simulink model "Controllerlogic"  (R2017a)
settings: Solver=ode23tb  StartTime=0.0  StopTime=Inf  RelTol=1e-4
libraries: dspnetwork x12, powerlib x8, sps_avr x7, simulink x3, dspstat3 x2, utility x1
Description:
  | Copyright 2008-2016 The MathWorks, Inc.
settings Model: FPTRunName=Active  ExtModeTrigMode=oneshot  ExtModeArmWhenConnect=off  ExtModeAutoUpdateStatusClock=off  Creator=MathWorks  LastModifiedBy=CCRE
settings SolverCC: ZeroCrossAlgorithm=Adaptive
settings DataIOCC: SaveFormat=Array  SignalLoggingSaveFormat=ModelDataLogs  SignalLoggingName=sigsOut  OutputTimes=[0:1/20:10]
settings OptimizationCC: BlockReduction=off  BooleanDataType=off  ExpressionDepthLimit=2147483647  InitFltsAndDblsToZero=on  EfficientMapNaN2IntZero=off  LifeSpan=inf
settings DebuggingCC: UnderspecifiedInitializationDetection=Classic  MergeDetectMultiDrivingBlocksExec=none  CheckExecutionContextPreStartOutputMsg=on  CheckExecutionContextRuntimeOutputMsg=on  SignalResolutionControl=TryResolveAllWithWarning  IgnoredZcDiagnostic=none  MultiTaskDSMMsg=warning  MultiTaskCondExecSysMsg=none  SigSpecEnsureSampleTimeMsg=none  FcnCallInpInsideContextMsg=warning  UnconnectedInputMsg=none  UnconnectedOutputMsg=none  UnconnectedLineMsg=none  StateNameClashWarn=warning  SFUnexpectedBacktrackingDiag=warning  SFNoUnconditionalDefaultTransitionDiag=warning  SFExecutionAtInitializationDiag=none
settings HardwareCC: ProdBitPerPointer=32  ProdBitPerSizeT=32  ProdBitPerPtrDiffT=32  ProdLargestAtomicFloat=None  ProdIntDivRoundTo=Undefined  ProdEndianess=Unspecified  ProdWordSize=32  ProdHWDeviceType=Specified  TargetUnknown=on
settings ModelReferenceCC: PropagateSignalLabelsOutOfModel=off
settings GRTTargetCC: TargetFcnLib=ansi_tfl_tmw.mat  TargetLangStandard=C89/C90 (ANSI)  GeneratePreprocessorConditionals=Disable all  CombineOutputUpdateFcns=off  GRTInterface=on
settings ConfigComp: CovMetricSettings=dw  CovHtmlReporting=on  CovSaveCumulativeToWorkspaceVar=on  CovSaveSingleToWorkspaceVar=on  CovExternalEMLEnable=off  CovSFcnEnable=off

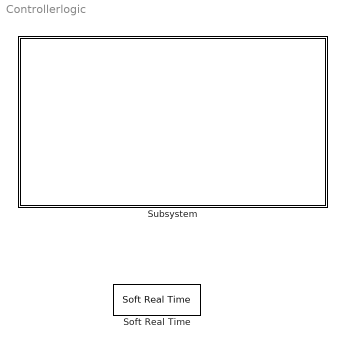
== system Controllerlogic ==
  Soft Real Time : utility/Soft Real Time  x=1
  Subsystem : Subsystem

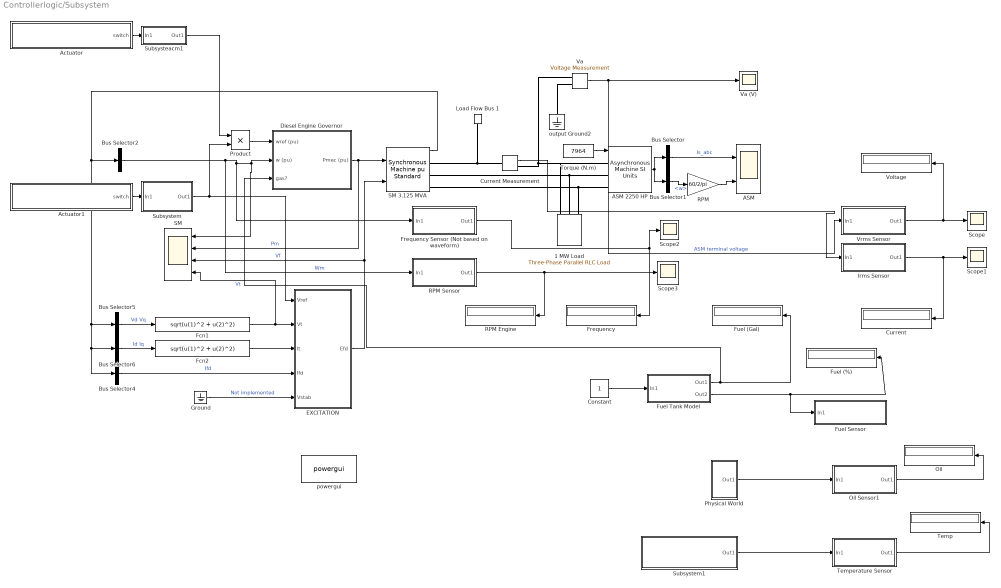
== system Controllerlogic/Subsystem ==
  1 MW Load : powerlib/Elements/Three-Phase Parallel RLC Load  LConnTagsString=A|B|C  Configuration=Y (grounded)  NominalVoltage=2400  Vabc=[1e3 1e3 1e3]  Vabcp=[1e3 1e3 1e3]  NominalFrequency=60  UnbalancedPower=off  ActivePower=1e+006  InductivePower=0  CapacitivePower=0  Pabc=[10e3 9e3 11e3]  QLabc=[100 90 110]  QCabc=[100 90 110]  Pabcp=[10e3 9e3 11e3]  QLabcp=[100 90 110]  QCabcp=[100 90 110]  Measurements=None  LoadType=constant Z
  ASM : Scope  NumInputPorts=2
  ASM 2250 HP : powerlib/Machines/Asynchronous Machine SI Units  RotorType=Squirrel-cage  PresetModel=No  MechanicalLoad=Torque Tm  ShowDetailedParameters=on  ReferenceFrame=Rotor  Units=SI  MeasurementBus=on  NominalParameters=[ 2250*746, 2400, 60 ]  Stator=[ 0.029 0.226/377]  Rotor=[ 0.022 0.226/377]  Cage1=[ 0.022 0.226/377]  Cage2=[ 0.022 0.226/377]  Lm=13.04/377  Mechanical=[ 63.87 0 2]  PolePairs=2  InitialConditions=[0 0 0 0 0 0 0 0]  SimulateSaturation=off  Saturation=[14.03593122, 27.81365428, 53.79336849, 72.68890987, 97.98006896, 148.6815601, 215.7428561, 302.9841135, 428.7778367 ; 230, 322, 414, 460, 506, 552, 598, 644, 690]  LoadFlowParameters=1492000  TsPowergui=0  TsBlock=-1  IterativeModel=Trapezoidal non iterative  IterativeDiscreteModel=Trapezoidal non iterative  Pmec=1.492e+006
  Actuator : Subsystem
  Actuator1 : Subsystem
  Bus Selector : BusSelector  OutputSignals=ias,ibs,ics  OutputAsBus=on
  Bus Selector1 : BusSelector  OutputSignals=w
  Bus Selector2 : BusSelector  OutputSignals="Mechanical.Rotor speed  wm  (pu)"  OutputAsBus=on
  Bus Selector4 : BusSelector  OutputSignals="dq0 components.Field current  ifd (pu)"  OutputAsBus=on
  Bus Selector5 : BusSelector  OutputSignals="dq0 components.Stator voltage  vd (pu),dq0 components.Stator voltage  vq (pu)"  OutputAsBus=on
  Bus Selector6 : BusSelector  OutputSignals="dq0 components.Stator current  id (pu),dq0 components.Stator current  iq (pu)"  OutputAsBus=on
  Constant : Constant
  Current : Display
  Current Measurement : powerlib/Measurements/Current Measurement  PhasorSimulation=off  OutputType=Complex  PSBequivalent=0
  "Diesel Engine Governor " : Subsystem  mask(Diesel Engine & Governor){K=1, Tr=[0.01 0.02 0.2], Ta=[0.25 0.009 0.0384], Tlim=[0 1.1], Td=0.024, Pm0=0}
      mask prompts: K "Regulator gain K:"; Tr "Regulator time constants [T1 T2 T3 ] (s) :"; Ta "Actuator time constants [T4 T5 T6] (s) :"; Tlim "Torque limits [Tmin Tmax] (pu) :"; Td "Engine time delay Td (s) :"; Pm0 "Initial value of mechanical power  Pm0 (pu) :"
      mask help:
      | This block implements a diesel engine and governor system:
      | 1st and 2nd inputs: Desired and actual speed (pu)
      | Output: Diesel engine mechanical power.Motor inertia should be combined with generator.
      | Controller transfer function:
      |      Hc=K.(1+T3.s)/(1+T1.s+T1.T2.s^2)
      | Actuator transfer function :
      |      Ha= (1+T4.s) / [ (s (1+T5.s)(1+T6.s) ]
      | Motor :
      |      Time delay Td
      |
      | (See reference in Tutorial Session 5)
  EXCITATION : Subsystem  Variant=on  OverrideUsingVariant=Variant1
      settings: AttributesFormatString=%<BlockChoice>
  Fcn1 : Fcn  Expr=sqrt(u(1)^2 + u(2)^2)
  Fcn2 : Fcn  Expr=sqrt(u(1)^2 + u(2)^2)
  Frequency : Display
  Frequency Sensor (Not based on waveform) : Subsystem
  Fuel (%) : Display
  Fuel (Gal) : Display
  Fuel Sensor : Subsystem
  Fuel Tank Model : Subsystem
  Ground : Ground
  Irms Sensor : Subsystem
  Load Flow Bus 1 : powerlib/Measurements/Load Flow Bus  LConnTagsString=a  Phases=single  Connectors=on one side  ID=B2  Vbase=2.4e3  Vref=1  Vangle=0  VLF=1  VLFb=1  VLFc=1  angleLF=-31.89  angleLFb=0  angleLFc=0
      settings: AttributesFormatString=%<ID>\n%<Vbase>V\n%<VLF>pu\n%<angleLF>deg.  SourceProductName=Simscape Power Systems
  Oil : Display
  Oil Sensor1 : Subsystem
  Physical World : Subsystem
  Product : Product
  RPM : Gain  Gain=60/2/pi  SaturateOnIntegerOverflow=on  OutDataTypeStr=Inherit: Same as input  ParamDataTypeStr=Inherit: Same as input
  RPM Engine : Display
  RPM Sensor : Subsystem
  SM : Scope  NumInputPorts=4
  SM 3.125 MVA : powerlib/Machines/Synchronous Machine pu Standard  PresetModel=No  MechanicalLoad=Mechanical power Pm  ShowDetailedParameters=on  RotorType=Salient-pole  Units=per unit standard parameters  MeasurementBus=off  NominalParameters="[ 3.125e6  2400  60]"  Reactances1=[ 31 32 33 34 35 36 37 ]  Reactances2=[ 1.56, 0.296, 0.177, 1.06, 0.177, 0.052 ]  dAxisTimeConstants=Short-circuit  qAxisTimeConstants=Open-circuit  TimeConstants1=[]  TimeConstants2=[]  TimeConstants3=[]  TimeConstants4=[]  TimeConstants5=[ 3.7, 0.05, 0.05 ]  TimeConstants6=[ 8.0, 0.03, 0.3371, 0.0295 ]  TimeConstants7=[0.024 0.006 0.006]  TimeConstants8=[]  StatorResistance=0.0036  Mechanical="[ 1.07  0 2]"  PolePairs=2  InitialConditions=[0 0 0 0 0 0 0 0 1]  SetSaturation=off  Saturation=[0.211 0.418 1.0 1.25 1.72 3.35 ;0.25 0.50 1.0 1.1 1.2 1.4]  LoadFlowParameters=[1 0 0 0]  TsPowergui=0  TsBlock=-1  IterativeModel=Trapezoidal non iterative  IterativeDiscreteModel=Trapezoidal non iterative  BusType=PV  Pref=0  Qref=0  Qmin=-Inf  Qmax=Inf  PLF=0  QLF=0
      settings: AttributesFormatString=\n\n  SourceProductName=Simscape Power Systems
  Scope{,1..3} (4 alike) : Scope
  Subsysteacm1 : Subsystem
  Subsystem : Subsystem
  Subsystem1 : Subsystem
  Temp : Display
  Temperature Sensor : Subsystem
  Torque (N.m) : Constant  Value=7964
  Va : powerlib/Measurements/Voltage Measurement  Tag=PoWeRsYsTeMmEaSuReMeNt  PhasorSimulation=off  OutputType=Magnitude  PSBequivalent=0
  Va (V) : Scope
  Voltage : Display
  Vrms Sensor : Subsystem
  output Ground2 : powerlib/Elements/Ground  LConnTagsString=a
  powergui : powerlib/powergui  Priority=2  SimulationMode=Continuous  SampleTime=50e-6  frequency=60  Iterations=50  frequencyindice=60  Pbase=1e6  ErrMax=0.0001  UnitsV=kV  UnitsW=MW  buscounter=0  FunctionMessages=off  echomessages=off  EnableUseOfTLC=off  CurrentSourceSwitches=off  DisableSnubberDevices=on  DisableRonSwitches=off  DisableVfSwitches=off  DisplayEquations=off  SolverType=Tustin  Interpol=off  ExternalGateDelay=off  methode=off  Ts=0  x0status=blocks  SPID=on  SwTol=0  HookPort=off  RestoreLinks=warning  ResistiveCurrentMeasurement=off  Frange=logspace(0,3,50)  Ylog=off  Xlog=off  ShowGrid=off  save=off  variable=ZData  structure=0  ZoomFFT=on  StartTime=0.0  cycles=2  DisplayStyle=off  fundamental=60  FreqAxis=off  MaxFrequency=1000  frequencyindicesteady=1  RmsSteady=1  display=off
  wires:
  "Diesel Engine Governor "/1(Pmec (pu)) -> SM/2, SM 3.125 MVA/1  "Pm"
  Bus Selector4/1 -> EXCITATION/4(Ifd)  "Ifd"
  Bus Selector5/1 -> Fcn1/1  "Vd Vq"
  Bus Selector2/1 -> RPM Sensor/1(In1), Frequency Sensor (Not based on waveform)/1(In1), SM/1, "Diesel Engine Governor "/2(w (pu))  "Wm"
  Bus Selector1/1 -> RPM/1  "<w>"
  Fcn1/1 -> SM/4, EXCITATION/2(Vt)  "Vt"
  RPM/1 -> ASM/2
  Bus Selector6/1 -> Fcn2/1  "Id Iq"
  Ground/1 -> EXCITATION/5(Vstab)  "Not implemented"
  Bus Selector/1 -> ASM/1  "Is_abc"
  Fcn2/1 -> EXCITATION/3(It)
  EXCITATION/1(Efd) -> SM 3.125 MVA/2, SM/3  "Vf"
  SM 3.125 MVA/1 -> Bus Selector5/1, Bus Selector6/1, Bus Selector4/1, Bus Selector2/1
  Vrms Sensor/1(Out1) -> Voltage/1, Scope/1
  Irms Sensor/1(Out1) -> Current/1, Scope1/1
  Va/1 -> Vrms Sensor/1(In1), Va (V)/1  "ASM terminal voltage"
  Current Measurement/1 -> Irms Sensor/1(In1)
  ASM 2250 HP/1 -> Bus Selector/1, Bus Selector1/1
  Torque (N.m)/1 -> ASM 2250 HP/1
  RPM Sensor/1(Out1) -> Scope3/1, RPM Engine/1
  Frequency Sensor (Not based on waveform)/1(Out1) -> Scope2/1, Frequency/1
  Constant/1 -> Fuel Tank Model/1(In1)
  Fuel Tank Model/2(Out2) -> Fuel Sensor/1(In1), Fuel (%)/1
  Product/1 -> "Diesel Engine Governor "/1(wref (pu))
  Oil Sensor1/1(Out1) -> Oil/1
  Subsystem/1(Out1) -> EXCITATION/1(Vref), Product/2
  Actuator1/1("switch ") -> Subsystem/1(In1)
  Temperature Sensor/1(Out1) -> Temp/1
  Actuator/1("switch ") -> Subsysteacm1/1(In1)
  Subsysteacm1/1(Out1) -> Product/1
  Fuel Tank Model/1(Out1) -> "Diesel Engine Governor "/3(gas?), Fuel (Gal)/1
  Physical World/1(Out1) -> Oil Sensor1/1(In1)
  Subsystem1/1(Out1) -> Temperature Sensor/1(In1)
  connections:
  SM 3.125 MVA/RConn3 -- ASM 2250 HP/LConn3 -- 1 MW Load/LConn3
  ASM 2250 HP/LConn1 -- 1 MW Load/LConn1 -- Current Measurement/RConn1 -- Va/LConn1
  output Ground2/LConn1 -- Va/LConn2
  SM 3.125 MVA/RConn2 -- ASM 2250 HP/LConn2 -- 1 MW Load/LConn2
  Load Flow Bus 1/LConn1 -- Current Measurement/LConn1 -- SM 3.125 MVA/RConn1

== system Controllerlogic/Subsystem/Actuator ==
  note: Pump Control
  Display : Display
  Pump If : If  IfExpression=u1 == 0
  Pump Value Conversion : Subsystem  TreatAsAtomicUnit=on
  Terminator : Terminator
  Terminator2 : Terminator
  UDP Receive1 : dspnetwork/UDP Receive  localURL='0.0.0.0'  localPort=10006  remoteURL='0.0.0.0'  remotePort=-1  recvBufferSize=8192  dims=1  signalDatatype=uint8  isVarSize=off  showBlockingTime=on  blockingTime=0  sampletime=0.01  blockPlatform=LINUX
  "switch " : Outport  PortDimensions=1
  wires:
  Pump If/1 -> Terminator/1
  Pump If/2 -> Pump Value Conversion/Action
  UDP Receive1/1 -> Pump Value Conversion/1(P_ASCII), Pump If/1
  Pump Value Conversion/1(P_Val) -> "switch "/1, Display/1
  UDP Receive1/2 -> Terminator2/1

== system Controllerlogic/Subsystem/Actuator1 ==
  note: Pump Control
  Display : Display
  Pump If : If  IfExpression=u1 == 0
  Pump Value Conversion : Subsystem  TreatAsAtomicUnit=on
  Terminator : Terminator
  Terminator2 : Terminator
  UDP Receive1 : dspnetwork/UDP Receive  localURL='0.0.0.0'  localPort=10007  remoteURL='0.0.0.0'  remotePort=-1  recvBufferSize=8192  dims=1  signalDatatype=uint8  isVarSize=off  showBlockingTime=on  blockingTime=0  sampletime=0.01  blockPlatform=LINUX
  "switch " : Outport  PortDimensions=1
  wires:
  Pump If/1 -> Terminator/1
  Pump If/2 -> Pump Value Conversion/Action
  UDP Receive1/1 -> Pump Value Conversion/1(P_ASCII), Pump If/1
  Pump Value Conversion/1(P_Val) -> "switch "/1, Display/1
  UDP Receive1/2 -> Terminator2/1

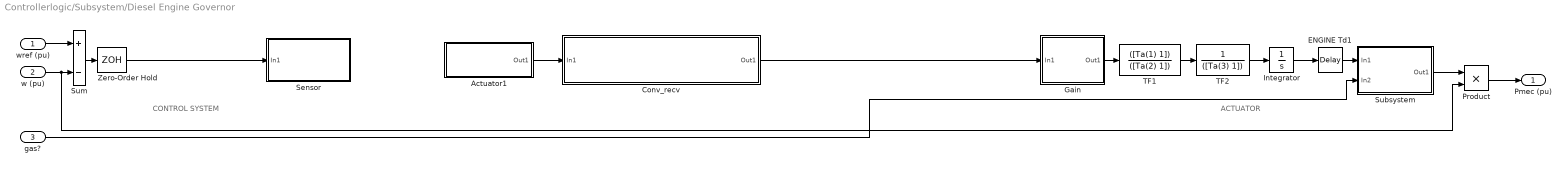
== system Controllerlogic/Subsystem/Diesel Engine Governor  ==
  note: ACTUATOR
  note: CONTROL SYSTEM
  wref (pu) : Inport
  w (pu) : Inport  Port=2
  gas? : Inport  Port=3
  Actuator1 : Subsystem
  Conv_recv : Subsystem
  ENGINE Td1 : TransportDelay  DelayTime=Td  InitialOutput=Pm0
  Gain : Subsystem
  Integrator : Integrator  InitialCondition=Pm0  LimitOutput=on  UpperSaturationLimit=Tlim(2)  LowerSaturationLimit=Tlim(1)
  Product : Product  SaturateOnIntegerOverflow=on  InputSameDT=on  OutDataTypeStr=Inherit: Same as first input
  Sensor : Subsystem
  Subsystem : Subsystem
  Sum : Sum  Inputs=+-  SaturateOnIntegerOverflow=on  InputSameDT=on  OutDataTypeStr=Inherit: Same as first input
  TF1 : TransferFcn  Numerator=([Ta(1) 1])  Denominator=([Ta(2) 1])
  TF2 : TransferFcn  Numerator=1  Denominator=([Ta(3) 1])
  Zero-Order Hold : ZeroOrderHold  SampleTime=.02
  Pmec (pu) : Outport  InitialOutput=0
  wires:
  Product/1 -> Pmec (pu)/1
  wref (pu)/1 -> Sum/1
  w (pu)/1 -> Sum/2, Product/2
  TF1/1 -> TF2/1
  Sum/1 -> Zero-Order Hold/1
  gas?/1 -> Subsystem/2(In2)
  TF2/1 -> Integrator/1
  Integrator/1 -> ENGINE Td1/1
  Subsystem/1(Out1) -> Product/1
  ENGINE Td1/1 -> Subsystem/1(In1)
  Conv_recv/1(Out1) -> Gain/1(In1)
  Gain/1(Out1) -> TF1/1
  Zero-Order Hold/1 -> Sensor/1(In1)
  Actuator1/1(Out1) -> Conv_recv/1(In1)

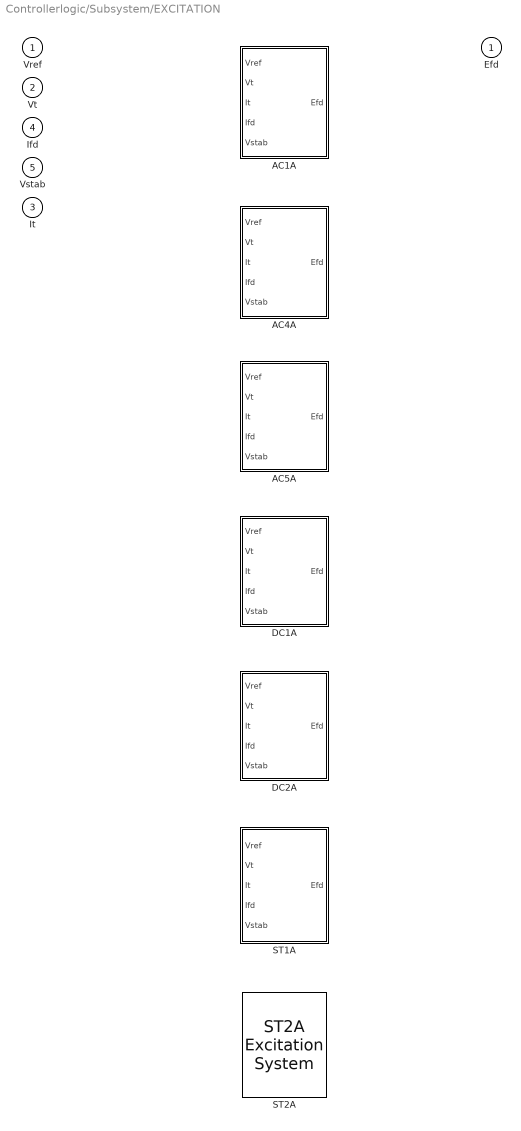
== system Controllerlogic/Subsystem/EXCITATION ==
  Vref : Inport
  Vt : Inport  Port=2
  It : Inport  Port=3
  Ifd : Inport  Port=4
  Vstab : Inport  Port=5
  AC1A : Subsystem  VariantControl=Variant1
  AC4A : Subsystem  VariantControl=Variant2
  AC5A : Subsystem  VariantControl=Variant3
  DC1A : Subsystem  VariantControl=Variant4
  DC2A : Subsystem  VariantControl=Variant5
  ST1A : Subsystem  VariantControl=Variant6
  ST2A : sps_avr/ST2A Excitation System  VariantControl=Variant7  Tr=20e-3  KaTa=[120 0.15]  VRminmax=[0 1.0]  KfTf=[0.05 1.0]  KeTe=[1.0 0.5]  KI=8.0  Kp=4.88  Xd=1.56  Kc=1.82  v0=[1,1.42734]  I0=0.2739  TsBlock=-2
      settings: SourceProductName=Simscape Power Systems  SourceProductBaseCode=PS
  Efd : Outport

== system Controllerlogic/Subsystem/Frequency Sensor (Not based on waveform) ==
  In1 : Inport
  Downsample : DownSample  N=100  RateOptions=Allow multirate processing
  Gain : Gain  Gain=6000
  UDP Send : dspnetwork/UDP Send  remoteURL='192.168.56.101'  remotePort=10003  localURL='255.255.255.255'  localPortSource=Automatically determine  localPort=-1  sampletime=-1  blockPlatform=LINUX  separateLengthPort=0
  Zero-Order Hold : ZeroOrderHold  SampleTime=.001
  Out1 : Outport
  wires:
  In1/1 -> Zero-Order Hold/1
  Zero-Order Hold/1 -> Gain/1
  Downsample/1 -> UDP Send/1, Out1/1
  Gain/1 -> Downsample/1

== system Controllerlogic/Subsystem/Fuel Sensor ==
  In1 : Inport
  Rate Transition : RateTransition
  UDP Send : dspnetwork/UDP Send  remoteURL='192.168.56.101'  remotePort=10005  localURL='255.255.255.255'  localPortSource=Automatically determine  localPort=-1  sampletime=-1  blockPlatform=LINUX  separateLengthPort=0
  Zero-Order Hold1 : ZeroOrderHold  SampleTime=0.1
  Zero-Order Hold2 : ZeroOrderHold  SampleTime=0.01
  wires:
  Rate Transition/1 -> Zero-Order Hold1/1
  Zero-Order Hold1/1 -> UDP Send/1
  Zero-Order Hold2/1 -> Rate Transition/1
  In1/1 -> Zero-Order Hold2/1

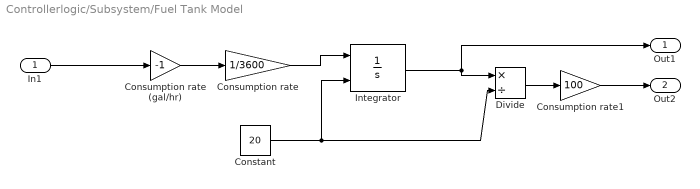
== system Controllerlogic/Subsystem/Fuel Tank Model ==
  In1 : Inport
  Constant : Constant  Value=20
  Consumption rate : Gain  Gain=1/3600
  Consumption rate (gal/hr) : Gain  Gain=-1
  Consumption rate1 : Gain  Gain=100
  Divide : Product  Inputs=*/
  Integrator : Integrator  InitialConditionSource=external  InitialCondition=20  LimitOutput=on  UpperSaturationLimit=20  LowerSaturationLimit=0
  Out1 : Outport
  Out2 : Outport  Port=2
  wires:
  In1/1 -> Consumption rate (gal/hr)/1
  Constant/1 -> Divide/2, Integrator/2
  Integrator/1 -> Divide/1, Out1/1
  Consumption rate1/1 -> Out2/1
  Divide/1 -> Consumption rate1/1
  Consumption rate (gal/hr)/1 -> Consumption rate/1
  Consumption rate/1 -> Integrator/1

== system Controllerlogic/Subsystem/Irms Sensor ==
  In1 : Inport
  Downsample : DownSample  N=100  RateOptions=Allow multirate processing
  RMS : dspstat3/RMS  run=on  directionMode=Entire input  dimension=1  reset_popup=None
  UDP Send : dspnetwork/UDP Send  remoteURL='192.168.56.101'  remotePort=10002  localURL='255.255.255.255'  localPortSource=Automatically determine  localPort=-1  sampletime=-1  blockPlatform=LINUX  separateLengthPort=0
  Zero-Order Hold : ZeroOrderHold  SampleTime=.001
  Out1 : Outport
  wires:
  In1/1 -> Zero-Order Hold/1
  RMS/1 -> Downsample/1
  Zero-Order Hold/1 -> RMS/1
  Downsample/1 -> Out1/1, UDP Send/1

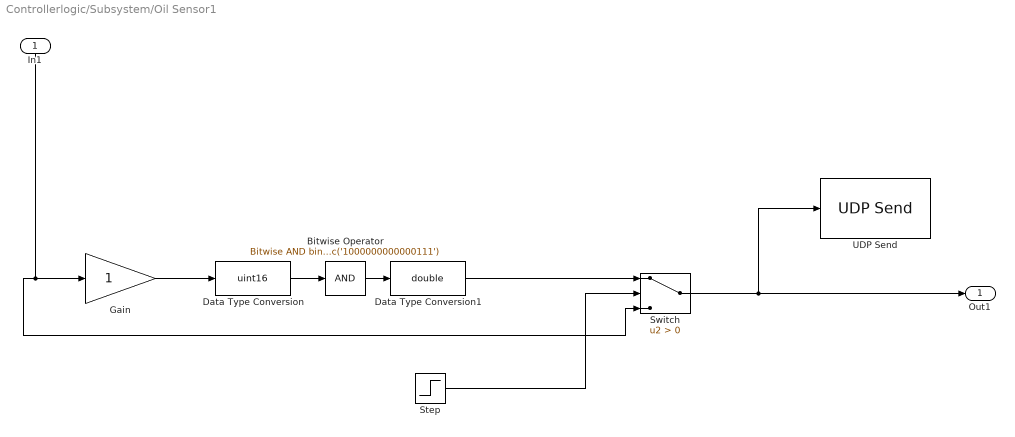
== system Controllerlogic/Subsystem/Oil Sensor1 ==
  In1 : Inport
  Bitwise Operator : simulink/Logic and Bit Operations/Bitwise Operator  logicop=AND  UseBitMask=on  BitMask=bin2dec('1000000000000111')  BitMaskRealWorld=Stored Integer
  Data Type Conversion : DataTypeConversion  OutDataTypeStr=uint16
  Data Type Conversion1 : DataTypeConversion  OutDataTypeStr=double
  Gain : Gain
  Step : Step  SampleTime=0
  Switch : Switch  Criteria=u2 > Threshold
  UDP Send : dspnetwork/UDP Send  remoteURL='192.168.56.101'  remotePort=10008  localURL='255.255.255.255'  localPortSource=Automatically determine  localPort=-1  sampletime=-1  blockPlatform=LINUX  separateLengthPort=0
  Out1 : Outport
  wires:
  In1/1 -> Gain/1, Switch/3
  Bitwise Operator/1 -> Data Type Conversion1/1
  Gain/1 -> Data Type Conversion/1
  Data Type Conversion/1 -> Bitwise Operator/1
  Switch/1 -> UDP Send/1, Out1/1
  Data Type Conversion1/1 -> Switch/1
  Step/1 -> Switch/2

== system Controllerlogic/Subsystem/Physical World ==
  Constant1 : Constant  Value=10
  Constant2 : Constant  Value=50
  Manual Switch : ManualSwitch
  Out1 : Outport
  wires:
  Constant2/1 -> Manual Switch/1
  Constant1/1 -> Manual Switch/2
  Manual Switch/1 -> Out1/1

== system Controllerlogic/Subsystem/RPM Sensor ==
  In1 : Inport
  Downsample : DownSample  N=100  RateOptions=Allow multirate processing
  Gain : Gain  Gain=3600
  UDP Send : dspnetwork/UDP Send  remoteURL='192.168.56.101'  remotePort=10004  localURL='255.255.255.255'  localPortSource=Automatically determine  localPort=-1  sampletime=-1  blockPlatform=LINUX  separateLengthPort=0
  Zero-Order Hold : ZeroOrderHold  SampleTime=.001
  Out1 : Outport
  wires:
  In1/1 -> Zero-Order Hold/1
  Zero-Order Hold/1 -> Gain/1
  Downsample/1 -> Out1/1, UDP Send/1
  Gain/1 -> Downsample/1

== system Controllerlogic/Subsystem/Subsysteacm1 ==
  In1 : Inport
  Switch : Switch  Criteria=u2 > Threshold
  wref (pu) : Constant  Value=50/60
  wref (pu)1 : Constant
  Out1 : Outport
  wires:
  wref (pu)/1 -> Switch/1
  In1/1 -> Switch/2
  Switch/1 -> Out1/1
  wref (pu)1/1 -> Switch/3

== system Controllerlogic/Subsystem/Subsystem ==
  In1 : Inport
  Subtract : Sum  Inputs=+-
  "Vtref (pu) " : Constant
  Out1 : Outport
  wires:
  Subtract/1 -> Out1/1
  In1/1 -> Subtract/2
  "Vtref (pu) "/1 -> Subtract/1

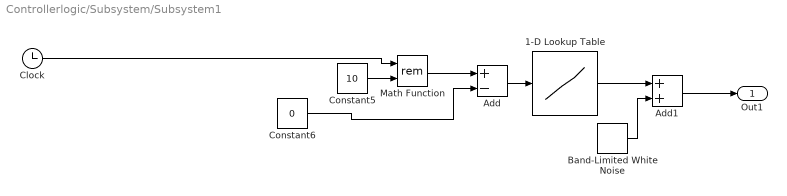
== system Controllerlogic/Subsystem/Subsystem1 ==
  1-D Lookup Table : Lookup_n-D  NumberOfTableDimensions=1  BreakpointsForDimension1=[0 1 2 3 4 5 6 7 8 9 10]  Table=[95 160 95 110 180 110 220 150 110 220 100]  InternalRulePriority=Speed  RndMeth=Simplest  InputSameDT=on
  Add : Sum  Inputs=+-
  Add1 : Sum
  Band-Limited White Noise : simulink/Sources/Band-Limited White Noise  Cov=[0.3]  Ts=0.02  seed=[23341]
  Clock : Clock
  Constant5 : Constant  Value=10
  Constant6 : Constant  Value=0
  Math Function : Math  Operator=rem  SaturateOnIntegerOverflow=on
  Out1 : Outport
  wires:
  Band-Limited White Noise/1 -> Add1/2
  Add/1 -> 1-D Lookup Table/1
  Constant6/1 -> Add/2
  Constant5/1 -> Math Function/2
  Math Function/1 -> Add/1
  Clock/1 -> Math Function/1
  Add1/1 -> Out1/1
  1-D Lookup Table/1 -> Add1/1

== system Controllerlogic/Subsystem/Temperature Sensor ==
  In1 : Inport
  Downsample : DownSample  N=100  RateOptions=Allow multirate processing
  Gain : Gain
  HW Trojan : Subsystem
  UDP Send : dspnetwork/UDP Send  remoteURL='192.168.56.101'  remotePort=10009  localURL='255.255.255.255'  localPortSource=Automatically determine  localPort=-1  sampletime=-1  blockPlatform=LINUX  separateLengthPort=0
  Zero-Order Hold : ZeroOrderHold  SampleTime=.001
  Out1 : Outport
  wires:
  In1/1 -> Zero-Order Hold/1
  Zero-Order Hold/1 -> Gain/1
  Downsample/1 -> HW Trojan/1(In1)
  Gain/1 -> Downsample/1
  HW Trojan/1(Out1) -> Out1/1, UDP Send/1

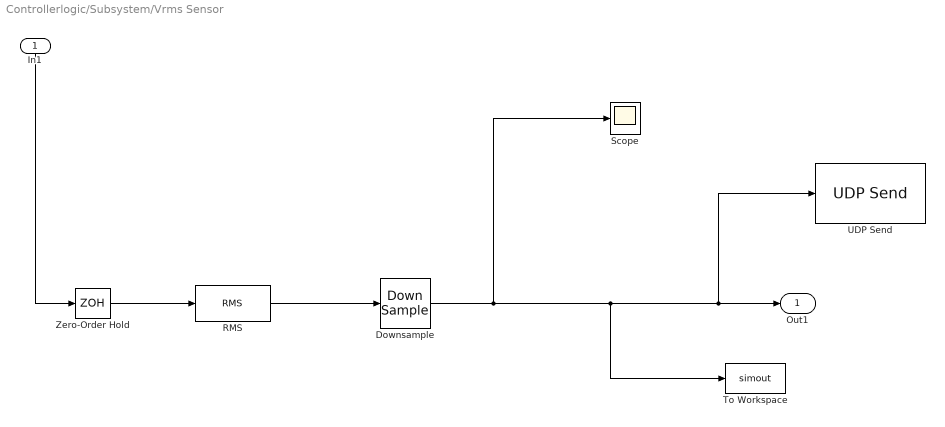
== system Controllerlogic/Subsystem/Vrms Sensor ==
  In1 : Inport
  Downsample : DownSample  N=100  RateOptions=Allow multirate processing
  RMS : dspstat3/RMS  run=on  directionMode=Entire input  dimension=1  reset_popup=None
  Scope : Scope
  To Workspace : ToWorkspace  VariableName=simout  SaveFormat=Timeseries  SampleTime=-1
  UDP Send : dspnetwork/UDP Send  remoteURL='192.168.56.101'  remotePort=10001  localURL='255.255.255.255'  localPortSource=Automatically determine  localPort=-1  sampletime=-1  blockPlatform=LINUX  separateLengthPort=0
  Zero-Order Hold : ZeroOrderHold  SampleTime=.001
  Out1 : Outport
  wires:
  In1/1 -> Zero-Order Hold/1
  Downsample/1 -> Scope/1, To Workspace/1, Out1/1, UDP Send/1
  RMS/1 -> Downsample/1
  Zero-Order Hold/1 -> RMS/1

== system Controllerlogic/Subsystem/Actuator/Pump Value Conversion ==
  P_ASCII : Inport
  Action Port : ActionPort  ActionType=else
  '0' : Constant  Value=48
  Subtract : Sum  Inputs=+-
  P_Val : Outport
  wires:
  P_ASCII/1 -> Subtract/1
  Subtract/1 -> P_Val/1
  '0'/1 -> Subtract/2

== system Controllerlogic/Subsystem/Actuator1/Pump Value Conversion ==
  P_ASCII : Inport
  Action Port : ActionPort  ActionType=else
  '0' : Constant  Value=48
  Subtract : Sum  Inputs=+-
  P_Val : Outport
  wires:
  P_ASCII/1 -> Subtract/1
  Subtract/1 -> P_Val/1
  '0'/1 -> Subtract/2

== system Controllerlogic/Subsystem/Diesel Engine Governor /Actuator1 ==
  To Workspace : ToWorkspace  VariableName=Act  SaveFormat=Timeseries  SampleTime=-1
  UDP Receive : dspnetwork/UDP Receive  localURL='0.0.0.0'  localPort=10003  remoteURL='0.0.0.0'  remotePort=-1  recvBufferSize=2  dims=1  signalDatatype=uint16  isVarSize=off  showBlockingTime=on  blockingTime=0  sampletime=-1  blockPlatform=LINUX
  Voltage1 : Display
  Voltage2 : Display
  Out1 : Outport
  wires:
  UDP Receive/2 -> Voltage2/1
  UDP Receive/1 -> Voltage1/1, Out1/1, To Workspace/1

== system Controllerlogic/Subsystem/Diesel Engine Governor /Conv_recv ==
  In1 : Inport
  Constant : Constant  Value=10000
  Constant1 : Constant  Value=10000
  Divide : Product  Inputs=*/
  Sum2 : Sum  Inputs=|+-
  Out1 : Outport
  wires:
  In1/1 -> Sum2/1
  Divide/1 -> Out1/1
  Sum2/1 -> Divide/1
  Constant/1 -> Sum2/2
  Constant1/1 -> Divide/2

== system Controllerlogic/Subsystem/Diesel Engine Governor /Gain ==
  In1 : Inport
  Custom Gain Actuator : Subsystem
  Gain K : Gain  Gain=-1  SaturateOnIntegerOverflow=on  OutDataTypeStr=Inherit: Same as input  ParamDataTypeStr=Inherit: Same as input
  Product1 : Product
  Out1 : Outport
  wires:
  In1/1 -> Gain K/1
  Custom Gain Actuator/1(Out1) -> Product1/2
  Product1/1 -> Out1/1
  Gain K/1 -> Product1/1

== system Controllerlogic/Subsystem/Diesel Engine Governor /Sensor ==
  In1 : Inport
  Conv_send : Subsystem
  Sensor : Subsystem
  wires:
  In1/1 -> Conv_send/1(In1)
  Conv_send/1(Out1) -> Sensor/1(In1)

== system Controllerlogic/Subsystem/Diesel Engine Governor /Subsystem ==
  In1 : Inport
  In2 : Inport  Port=2
  Ground : Ground
  Switch : Switch  Criteria=u2 > Threshold
  Out1 : Outport
  wires:
  Switch/1 -> Out1/1  "Torque"
  In1/1 -> Switch/1
  Ground/1 -> Switch/3
  In2/1 -> Switch/2

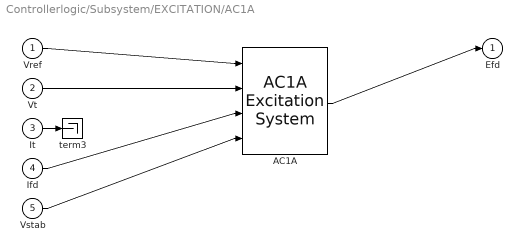
== system Controllerlogic/Subsystem/EXCITATION/AC1A ==
  Vref : Inport
  Vt : Inport  Port=2
  It : Inport  Port=3
  Ifd : Inport  Port=4
  Vstab : Inport  Port=5
  AC1A : sps_avr/AC1A Excitation System  Tr=20e-3  KaTa=[400 0.02]  VAminmax=[-14.5 14.5]  VRminmax=[-5.43 6.03]  KfTf=[0.03 1.0]  TbTc=[0 0]  KeTe=[1.0 0.80]  Ve12=[4.18 3.14]  SeVe12=[0.10 0.03]  Kd=0.38  Kc=0.20  v0=[1 1.4273]  TsBlock=-2
      settings: SourceProductName=Simscape Power Systems  SourceProductBaseCode=PS
  term3 : Terminator
  Efd : Outport
  wires:
  It/1 -> term3/1
  AC1A/1 -> Efd/1
  Vstab/1 -> AC1A/4
  Ifd/1 -> AC1A/3
  Vt/1 -> AC1A/2
  Vref/1 -> AC1A/1

== system Controllerlogic/Subsystem/EXCITATION/AC4A ==
  Vref : Inport
  Vt : Inport  Port=2
  It : Inport  Port=3
  Ifd : Inport  Port=4
  Vstab : Inport  Port=5
  AC4A : sps_avr/AC4A Excitation System  Tr=20e-3  KaTa=[200 0.015]  VIminmax=[-10 10]  VRminmax=[-4.53 5.64]  TbTc=[10 1.0]  Kc=0  v0=[1,1.42734]  TsBlock=-2
      settings: SourceProductName=Simscape Power Systems  SourceProductBaseCode=PS
  term3 : Terminator
  Efd : Outport
  wires:
  It/1 -> term3/1
  AC4A/1 -> Efd/1
  Vstab/1 -> AC4A/4
  Ifd/1 -> AC4A/3
  Vt/1 -> AC4A/2
  Vref/1 -> AC4A/1

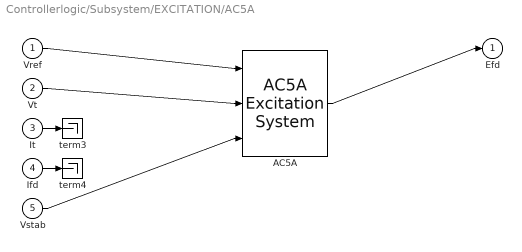
== system Controllerlogic/Subsystem/EXCITATION/AC5A ==
  Vref : Inport
  Vt : Inport  Port=2
  It : Inport  Port=3
  Ifd : Inport  Port=4
  Vstab : Inport  Port=5
  AC5A : sps_avr/AC5A Excitation System  Tr=20e-3  KaTa=[100 0.02]  VRminmax=[-7.3 7.3]  KfTf=[0.03 1 0 0]  KeTe=[1.0 0.02]  Efd12=[5.6 0.75*5.6]  SeEfd12=[0.86 0.5]  v0=[1,1.42734]  TsBlock=-2
      settings: SourceProductName=Simscape Power Systems  SourceProductBaseCode=PS
  term3 : Terminator
  term4 : Terminator
  Efd : Outport
  wires:
  Ifd/1 -> term4/1
  It/1 -> term3/1
  AC5A/1 -> Efd/1
  Vstab/1 -> AC5A/3
  Vt/1 -> AC5A/2
  Vref/1 -> AC5A/1

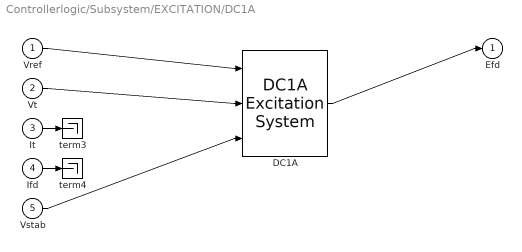
== system Controllerlogic/Subsystem/EXCITATION/DC1A ==
  Vref : Inport
  Vt : Inport  Port=2
  It : Inport  Port=3
  Ifd : Inport  Port=4
  Vstab : Inport  Port=5
  DC1A : sps_avr/DC1A Excitation System  Tr=20e-3  KaTa=[46 0.06]  VRminmax=[-0.9 1.0]  KfTf=[0.05 1.5]  TbTc=[0 0]  KeTe=[0.05 0.46]  Efd12=[3.1 2.3]  SeEfd12=[0.33 0.10]  v0=[1,1.42734]  TsBlock=-2
      settings: SourceProductName=Simscape Power Systems  SourceProductBaseCode=PS
  term3 : Terminator
  term4 : Terminator
  Efd : Outport
  wires:
  Ifd/1 -> term4/1
  It/1 -> term3/1
  DC1A/1 -> Efd/1
  Vstab/1 -> DC1A/3
  Vt/1 -> DC1A/2
  Vref/1 -> DC1A/1

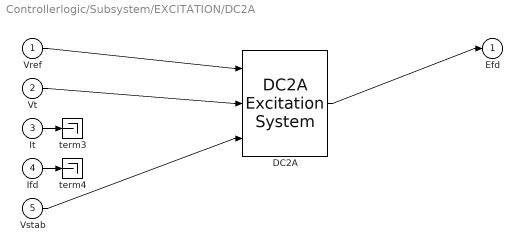
== system Controllerlogic/Subsystem/EXCITATION/DC2A ==
  Vref : Inport
  Vt : Inport  Port=2
  It : Inport  Port=3
  Ifd : Inport  Port=4
  Vstab : Inport  Port=5
  DC2A : sps_avr/DC2A Excitation System  Tr=20e-3  KaTa=[46 0.06]  VRminmax=[-4.9 4.95]  KfTf=[0.05 1.5]  TbTc=[0 0]  KeTe=[0.05 0.46]  Efd12=[3.05 2.29]  SeEfd12=[0.279 0.117]  v0=[1,1.42734]  TsBlock=-2
      settings: SourceProductName=Simscape Power Systems  SourceProductBaseCode=PS
  term3 : Terminator
  term4 : Terminator
  Efd : Outport
  wires:
  Ifd/1 -> term4/1
  It/1 -> term3/1
  DC2A/1 -> Efd/1
  Vstab/1 -> DC2A/3
  Vt/1 -> DC2A/2
  Vref/1 -> DC2A/1

== system Controllerlogic/Subsystem/EXCITATION/ST1A ==
  Vref : Inport
  Vt : Inport  Port=2
  It : Inport  Port=3
  Ifd : Inport  Port=4
  Vstab : Inport  Port=5
  ST1A : sps_avr/ST1A Excitation System  Tr=20e-3  KaTa=[210 0.001]  VIminmax=[-999 999]  VAminmax=[-999 999]  VRminmax=[-6.0 6.43]  KfTf=[0.001 1]  TbTc=[0 0 0 0]  KLR=1  ILR=2  Kc=0.038  v0=[1,1.42734]  TsBlock=-2
      settings: SourceProductName=Simscape Power Systems  SourceProductBaseCode=PS
  term3 : Terminator
  Efd : Outport
  wires:
  It/1 -> term3/1
  ST1A/1 -> Efd/1
  Vstab/1 -> ST1A/4
  Ifd/1 -> ST1A/3
  Vt/1 -> ST1A/2
  Vref/1 -> ST1A/1

== system Controllerlogic/Subsystem/Temperature Sensor/HW Trojan ==
  In1 : Inport
  Bitwise Operator : simulink/Logic and Bit Operations/Bitwise Operator  logicop=OR  UseBitMask=on  BitMask=bin2dec('0000111100000111')  BitMaskRealWorld=Stored Integer
  Data Type Conversion : DataTypeConversion  OutDataTypeStr=uint16
  Data Type Conversion1 : DataTypeConversion  OutDataTypeStr=double
  Gain1 : Gain
  Step : Step  Time=50  SampleTime=0
  Switch : Switch  Criteria=u2 > Threshold
  Out1 : Outport
  wires:
  In1/1 -> Switch/3, Gain1/1
  Data Type Conversion1/1 -> Switch/1
  Bitwise Operator/1 -> Data Type Conversion1/1
  Gain1/1 -> Data Type Conversion/1
  Step/1 -> Switch/2
  Data Type Conversion/1 -> Bitwise Operator/1
  Switch/1 -> Out1/1

== system Controllerlogic/Subsystem/Diesel Engine Governor /Gain/Custom Gain Actuator ==
  UDP Receive1 : dspnetwork/UDP Receive  localURL='0.0.0.0'  localPort=10011  remoteURL='0.0.0.0'  remotePort=-1  recvBufferSize=8192  dims=1  signalDatatype=uint16  isVarSize=off  showBlockingTime=on  blockingTime=0  sampletime=0.01  blockPlatform=LINUX
  Voltage1 : Display
  Voltage2 : Display
  Out1 : Outport
  wires:
  UDP Receive1/2 -> Voltage2/1
  UDP Receive1/1 -> Out1/1, Voltage1/1

== system Controllerlogic/Subsystem/Diesel Engine Governor /Sensor/Conv_send ==
  In1 : Inport
  Constant : Constant  Value=10000
  Constant1 : Constant  Value=10000
  Product1 : Product
  Sum1 : Sum  Inputs=|++
  Out1 : Outport
  wires:
  Product1/1 -> Sum1/1
  In1/1 -> Product1/1
  Sum1/1 -> Out1/1
  Constant1/1 -> Sum1/2
  Constant/1 -> Product1/2

== system Controllerlogic/Subsystem/Diesel Engine Governor /Sensor/Sensor ==
  In1 : Inport
  Scope : Scope
  To Workspace : ToWorkspace  VariableName=sen  SaveFormat=Timeseries  SampleTime=-1
  UDP Send : dspnetwork/UDP Send  remoteURL='192.168.56.101'  remotePort=10001  localURL='255.255.255.255'  localPortSource=Automatically determine  localPort=-1  sampletime=-1  blockPlatform=LINUX  separateLengthPort=0
  Zero-Order Hold : ZeroOrderHold  SampleTime=.01
  wires:
  In1/1 -> Zero-Order Hold/1
  Zero-Order Hold/1 -> Scope/1, To Workspace/1, UDP Send/1
